simulink model "TVCSimulationForMyModel"  (R2023a)
settings: Solver=VariableStepAuto  StartTime=0.0  StopTime=25  RelTol=1e-3
libraries: simulink x1, simulink_extras x1
settings Model: Creator=Administrator  LastModifiedBy=Administrator

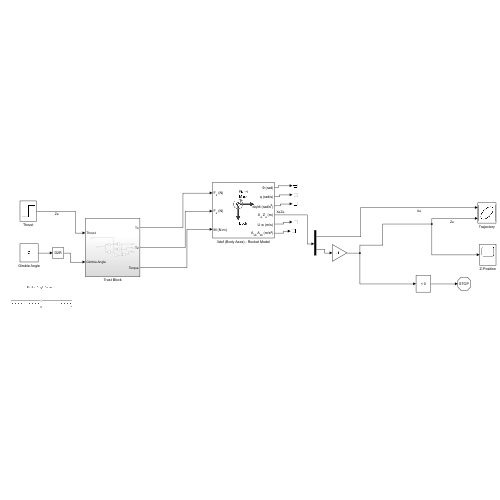
[thumbnail: Simulink's stored preview of the top-level diagram]
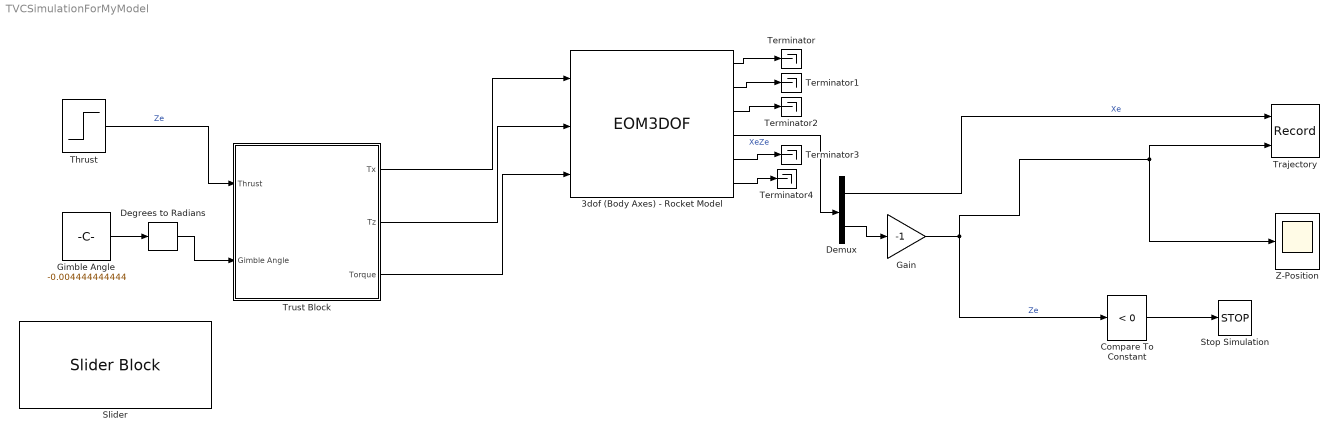
== system TVCSimulationForMyModel ==
  3dof (Body Axes) - Rocket Model : EOM3DOF  v_ini=0  mass=M_b  Iyy=MMOI
  Compare To Constant : simulink/Logic and Bit Operations/Compare To Constant  relop=<  const=0  OutDataTypeStr=boolean
  Degrees to Radians : simulink_extras/Transformations/Degrees to Radians
  Demux : Demux  Outputs=2
  Gain : Gain  Gain=-1
  Gimble Angle : Constant  Value=-0.004444444444
  Slider : SliderBlock  ScaleMin=-1  ScaleMax=1  TickInterval=1
  Stop Simulation : Stop
  Terminator{,1..4} (5 alike) : Terminator
  Thrust : Step  Time=2  Before=-30  After=0  SampleTime=0
  Trajectory : Record  FileSettingsInternal="{\"entries\":[{\"content\":{\"excelSettings\":{\"content\":{},\"type\":\"Streamout.ExcelSettings\"}},\"type\":\"Streamout.FileSettingStorage\",\"uuid\":\"2a76dd94-78ca-4cfb-9507-0577e1286062\"}],\"packageUris\":[\"http://schema.mathworks.com/mf0/streamout_blocks/R2020a\"],\"version\":\"1.0\"}"  Layout=[1 1]  SignalsInternal="{\"entries\":[{\"content\":{\"signals\":[{\"content\":{\"blockPath\":[\"TVCSimulationForMyModel/Trajectory\"],\"dimensions\":[1],\"domain\":\"TVCSimulationForMyModel/Trajectory\",\"lineColor\":\"#0072bd\",\"plots\":[1],\"port\":1,\"sid\":[\"\"],\"signalID\":950,\"signalName\":\"Xe\"},\"type\":\"RecordBlkView.Signal\",\"uuid\":\"66e8427e-6665-49b5-9898-e5458aba9632\"},{\"content\":{\"blockPath\":[\"TVCSimulationForMyModel/Trajectory\"],\"dimensions\":[1],\"domain\":\"TVCSimulationForMyModel/Trajectory\",\"lineColor\":\"#d95319\",\"plots\":[1],\"port\":2,\"sid\":[\"\"],\"signalID\":954,\"signalName\":\"Ze\"},\"type\":\"RecordBlkView.Signal\",\"uuid\":\"bb438045-2a61-476d-89dc-9110c6c0a2b1\"}]},\"type\":\"RecordBlkView.InputSignals\",\"uuid\":\"0b709722-06a2-4c61-841e-2f9221395c84\"}],\"packageUris\":[\"http://schema.mathworks.com/mf0/streamout_blocks/R2020a\"],\"version\":\"1.0\"}"  VisualizationBindings="{\"xyplotplugin\":{\"info\":[{\"series\":[{\"bindingParametersList\":[{\"parameter\":\"X-Axis\",\"signalID\":950,\"signalName\":\"Xe\"},{\"parameter\":\"Y-Axis\",\"signalID\":954,\"signalName\":\"Ze\"}],\"seriesID\":47153}],\"subplotID\":1}]}}"  CompatibilityTag=XY
  Trust Block : Subsystem
  Z-Position : Scope
  wires:
  3dof (Body Axes) - Rocket Model/4 -> Demux/1  "XeZe"
  Demux/2 -> Gain/1
  Gain/1 -> Compare To Constant/1, Z-Position/1, Trajectory/2  "Ze"
  Demux/1 -> Trajectory/1  "Xe"
  Compare To Constant/1 -> Stop Simulation/1
  Gimble Angle/1 -> Degrees to Radians/1
  Thrust/1 -> Trust Block/1(Thrust)  "Ze"
  Degrees to Radians/1 -> Trust Block/2(Gimble Angle)
  Trust Block/1(Tx) -> 3dof (Body Axes) - Rocket Model/1
  Trust Block/2(Tz) -> 3dof (Body Axes) - Rocket Model/2
  Trust Block/3(Torque) -> 3dof (Body Axes) - Rocket Model/3
  3dof (Body Axes) - Rocket Model/1 -> Terminator/1
  3dof (Body Axes) - Rocket Model/2 -> Terminator1/1
  3dof (Body Axes) - Rocket Model/3 -> Terminator2/1
  3dof (Body Axes) - Rocket Model/5 -> Terminator3/1
  3dof (Body Axes) - Rocket Model/6 -> Terminator4/1

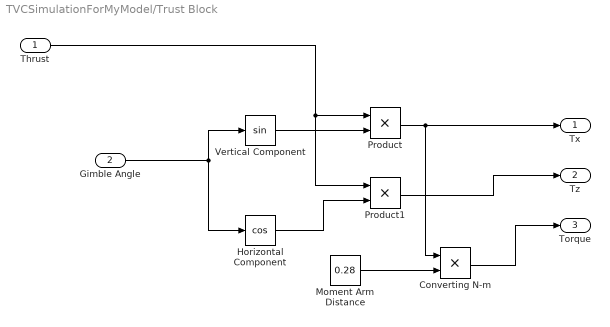
== system TVCSimulationForMyModel/Trust Block ==
  Thrust : Inport
  Gimble Angle : Inport  Port=2
  Converting N-m : Product
  Horizontal Component : Trigonometry  Operator=cos
  Moment Arm Distance : Constant  Value=0.28
  Product : Product
  Product1 : Product
  Vertical Component : Trigonometry
  Tx : Outport
  Tz : Outport  Port=2
  Torque : Outport  Port=3
  wires:
  Gimble Angle/1 -> Horizontal Component/1, Vertical Component/1
  Product/1 -> Tx/1, Converting N-m/1
  Converting N-m/1 -> Torque/1
  Thrust/1 -> Product1/1, Product/1
  Moment Arm Distance/1 -> Converting N-m/2
  Vertical Component/1 -> Product/2
  Product1/1 -> Tz/1
  Horizontal Component/1 -> Product1/2
